simulink model "controle_fuzzy"  (R2020a)
settings: Solver=VariableStepAuto  StartTime=0.0  StopTime=10.0  RelTol=1e-3
libraries: fuzblock x1
settings Model: Creator=Diego  LastModifiedBy=Diego

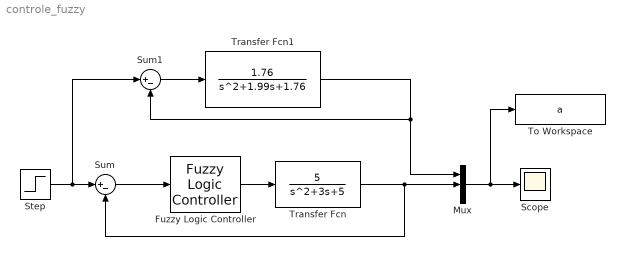
== system controle_fuzzy ==
  Fuzzy Logic Controller : fuzblock/Fuzzy Logic  Controller  FIS='controlador_fuzzy.fis'  OutputSampleNumber=101  DataType=double  FuzzifiedInputs=off  RuleFiringStrengths=off  RuleOutputs=off  AggregatedOutputs=off  SimulateUsing=Interpreted execution  OutOfRangeInputValueMessage=warning  NoRuleFiredMessage=warning  EmptyOutputFuzzySetMessage=warning
  Mux : Mux  Inputs=3
  Scope : Scope
  Step : Step  SampleTime=0
  Sum : Sum  Inputs=|+-
  Sum1 : Sum  Inputs=|+-
  To Workspace : ToWorkspace  VariableName=a  SaveFormat=Timeseries  SampleTime=-1
  Transfer Fcn : TransferFcn  Numerator=[5]  Denominator=[1 3 5]
  Transfer Fcn1 : TransferFcn  Numerator=[1.76]  Denominator=[1 1.99 1.76]
  wires:
  Transfer Fcn/1 -> Sum/2, Mux/2
  Step/1 -> Sum1/1, Sum/1
  Transfer Fcn1/1 -> Sum1/2, Mux/1
  Fuzzy Logic Controller/1 -> Transfer Fcn/1
  Sum/1 -> Fuzzy Logic Controller/1
  Mux/1 -> To Workspace/1, Scope/1
  Sum1/1 -> Transfer Fcn1/1
